simulink model "Sim_Forxards"  (R2019b)
settings: Solver=VariableStepAuto  StartTime=0.0  StopTime=10.0  RelTol=1e-3
values from neighbouring files (symbols this model uses):
  A = zeros(4,4)    [SP_Forwards.m]    (also in SP_Forwards_FH.m; SP_Sideways.m)
  B = zeros(4,1)    [SP_Forwards.m]    (also in SP_Forwards_FH.m; SP_Sideways.m)
  C = zeros(2,4)    [SP_Forwards.m]    (also in SP_Forwards_FH.m; SP_Sideways.m)
  D = zeros(2,1)    [SP_Forwards.m]    (also in SP_Forwards_FH.m; SP_Sideways.m)
  x0 = X0(1)    [SolveFODERK4.m]    (also in SolveSODERK4.m = X0(2))
undefined symbols (not defined in the file or in its folder): Discrete, K, Time
libraries: dspmtrx3 x1, ctrlSharedLib x1
settings Model: Creator=sam  LastModifiedBy=sam

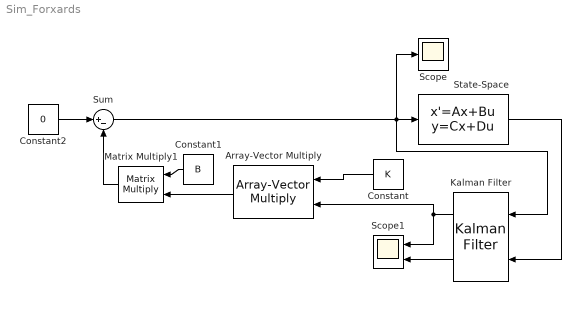
== system Sim_Forxards ==
  Array-Vector Multiply : dspmtrx3/Array-Vector Multiply  mode=Mute  saveAsFlag=0  Dimension=2  V_Source=Input port  V_VectFromMask=[0.5 0.25]  roundingMode=Floor  overflowMode=off  firstCoeffSignedness=Auto  firstCoeffDataTypeStr=Inherit: Same word length as input  firstCoeffMin=[]  firstCoeffMax=[]  firstCoeffLastDataTypeStr=Inherit: Same word length as input  prodOutputSignedness=Auto  accumSignedness=Auto  outputSignedness=Auto  outputDataTypeStr=Inherit: Same as product output  outputMin=[]  outputMax=[]  outputLastDataTypeStr=Inherit: Same as product output
      settings: SourceProductName=DSP System Toolbox  SourceProductBaseCode=DS
  Constant : Constant  Value=K
  Constant1 : Constant  Value=B
  Constant2 : Constant  Value=0
  Kalman Filter : ctrlSharedLib/Kalman Filter  TimeDomain=Discrete-Time  UseCurrentEstimator=on  ModelSource=LTI State-Space Variable  ModelSourceVariable=dt_sys  A=0.95  B=1  C=1  D=0  NumberOfStates=1  NumberOfInputs=1  NumberOfOutputs=1  InitialEstimateSource=Dialog  X0=x0  P0=10  UseK=off  UseGH=off  NumberOfProcessNoiseInputs=1  G=1  TimeInvariantG=on  H=0  TimeInvariantH=on  Q=0.05  TimeInvariantQ=on  R=1  TimeInvariantR=on  N=0  TimeInvariantN=on  AddInputPort=on  AddEnablePort=off  OutputEstimatedY=off  OutputP=on  Ts=-1
      settings: SourceProductBaseCode=CT
  Matrix Multiply1 : Product  Multiplication=Matrix(*)
  Scope : Scope
  Scope1 : Scope  NumInputPorts=2
  State-Space : StateSpace  A=A  B=B  C=C  D=D  InitialCondition=x0
  Sum : Sum  Inputs=|+-
  wires:
  State-Space/1 -> Kalman Filter/2
  Kalman Filter/1 -> Array-Vector Multiply/2, Scope1/1
  Sum/1 -> Scope/1, State-Space/1, Kalman Filter/1
  Array-Vector Multiply/1 -> Matrix Multiply1/2
  Constant1/1 -> Matrix Multiply1/1
  Matrix Multiply1/1 -> Sum/2
  Constant2/1 -> Sum/1
  Kalman Filter/2 -> Scope1/2
  Constant/1 -> Array-Vector Multiply/1
